simulink model "SimulacionControlador"  (R2023a)
settings: Solver=VariableStepAuto  StartTime=0.0  StopTime=5.0  RelTol=1e-3
settings Model: Creator=camil  LastModifiedBy=daniv

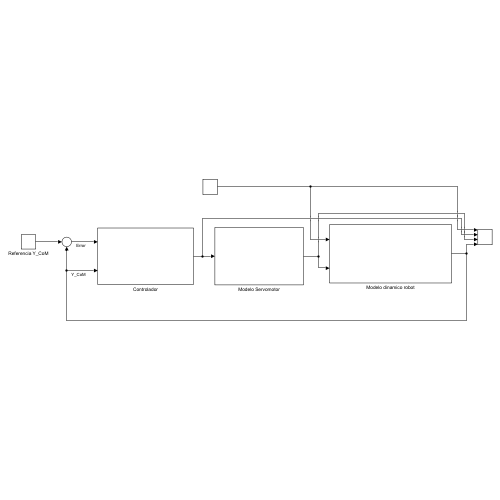
[thumbnail: Simulink's stored preview of the top-level diagram]
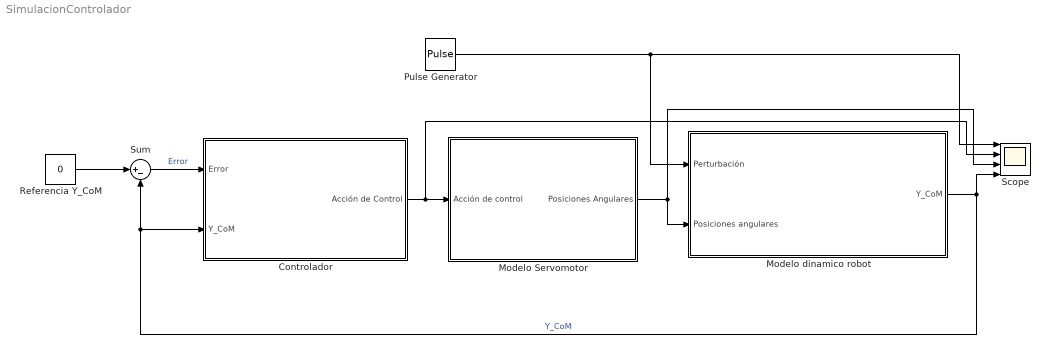
== system SimulacionControlador ==
  Controlador : Subsystem
  Modelo Servomotor : Subsystem
  Modelo dinamico robot : Subsystem
  Pulse Generator : DiscretePulseGenerator  PulseType=Time based  Amplitude=20  PulseWidth=50  PhaseDelay=1
  Referencia Y_CoM : Constant  Value=0
  Scope : Scope  NumInputPorts=4
  Sum : Sum  Inputs=|+-
  wires:
  Referencia Y_CoM/1 -> Sum/1
  Modelo Servomotor/1(Posiciones Angulares) -> Scope/3, Modelo dinamico robot/2(Posiciones angulares)
  Pulse Generator/1 -> Scope/1, Modelo dinamico robot/1(Perturbación)
  Controlador/1(Acción de Control) -> Scope/2, Modelo Servomotor/1(Acción de control)
  Sum/1 -> Controlador/1(Error)  "Error"
  Modelo dinamico robot/1(Y_CoM) -> Sum/2, Controlador/2(Y_CoM), Scope/4  "Y_CoM"

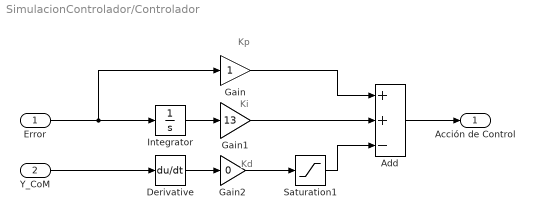
== system SimulacionControlador/Controlador ==
  note: Kd
  note: Ki
  note: Kp
  Error : Inport
  Y_CoM : Inport  Port=2
  Add : Sum  Inputs=++-
  Derivative : Derivative
  Gain : Gain
  Gain1 : Gain  Gain=13
  Gain2 : Gain  Gain=0
  Integrator : Integrator
  Saturation1 : Saturate  UpperLimit=10  LowerLimit=-10
  Acción de Control : Outport
  wires:
  Derivative/1 -> Gain2/1
  Add/1 -> Acción de Control/1
  Error/1 -> Integrator/1, Gain/1
  Saturation1/1 -> Add/3
  Gain/1 -> Add/1
  Gain1/1 -> Add/2
  Integrator/1 -> Gain1/1
  Y_CoM/1 -> Derivative/1
  Gain2/1 -> Saturation1/1

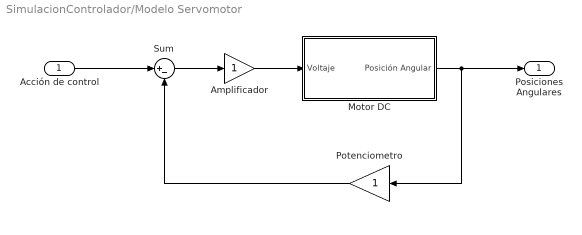
== system SimulacionControlador/Modelo Servomotor ==
  Acción de control : Inport
  Amplificador : Gain
  Motor DC : Subsystem
  Potenciometro : Gain
  Sum : Sum  Inputs=|+-
  Posiciones Angulares : Outport
  wires:
  Motor DC/1(Posición Angular) -> Posiciones Angulares/1, Potenciometro/1
  Acción de control/1 -> Sum/1
  Sum/1 -> Amplificador/1
  Potenciometro/1 -> Sum/2
  Amplificador/1 -> Motor DC/1(Voltaje)

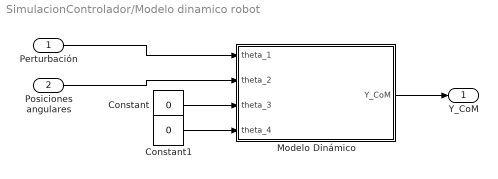
== system SimulacionControlador/Modelo dinamico robot ==
  Perturbación : Inport
  Posiciones angulares : Inport  Port=2
  Constant : Constant  Value=0
  Constant1 : Constant  Value=0
  Modelo Dinámico : MATLAB Function  TreatAsAtomicUnit=on
  Y_CoM : Outport
  wires:
  Perturbación/1 -> Modelo Dinámico/1(theta_1)
  Constant1/1 -> Modelo Dinámico/4(theta_4)
  Constant/1 -> Modelo Dinámico/3(theta_3)
  Modelo Dinámico/1(Y_CoM) -> Y_CoM/1
  Posiciones angulares/1 -> Modelo Dinámico/2(theta_2)

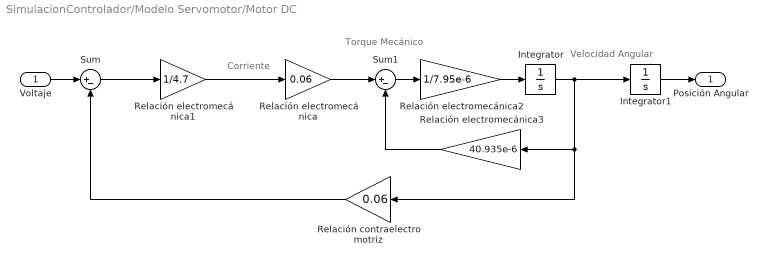
== system SimulacionControlador/Modelo Servomotor/Motor DC ==
  note: Torque
      | Mecánico
  note: Corriente
  note: Velocidad
      | Angular
  Voltaje : Inport
  Integrator : Integrator
  Integrator1 : Integrator
  Relación contraelectromotriz : Gain  Gain=0.06
  Relación electromecánica : Gain  Gain=0.06
  Relación electromecánica1 : Gain  Gain=1/4.7
  Relación electromecánica2 : Gain  Gain=1/7.95e-6
  Relación electromecánica3 : Gain  Gain=40.935e-6
  Sum : Sum  Inputs=|+-
  Sum1 : Sum  Inputs=|+-
  Posición Angular : Outport
  wires:
  Relación electromecánica3/1 -> Sum1/2
  Relación electromecánica2/1 -> Integrator/1
  Sum1/1 -> Relación electromecánica2/1
  Sum/1 -> Relación electromecánica1/1
  Relación electromecánica1/1 -> Relación electromecánica/1
  Relación contraelectromotriz/1 -> Sum/2
  Integrator/1 -> Integrator1/1, Relación electromecánica3/1, Relación contraelectromotriz/1
  Relación electromecánica/1 -> Sum1/1
  Voltaje/1 -> Sum/1
  Integrator1/1 -> Posición Angular/1

== matlab function SimulacionControlador/Modelo dinamico robot/Modelo Dinámico ==
  data: theta_1 input; Y_CoM output; theta_2 input; theta_3 input; theta_4 input
function Y_CoM = fcn(theta_1, theta_2, theta_3, theta_4)

% Vector de posiciones angulares
theta = [theta_1, theta_2, theta_3, theta_4];

% Vector de longitudes
L = [4, 24.5, 29, 11];

% Vector de posiciones de articulaciones
x = [0, 0, 0, 0];

% Calculo de posiciones de articulaciones
theta_sum = 0;
x_ant = 0;
for i = 1:length(theta)
        
    %Posicion x anterior
    if i == 1
        x_ant = 0;
    else 
        x_ant = x(i-1);
    end
    
    %Sumatoria de angulos
    for j = 1:i
        theta_sum = theta_sum + theta(i);
    end
    
    x(i) = x_ant + L(i)*sin((pi*theta_sum)/180);
end

% Vector de pesos
weight = [500, 334, 500, 330];

% Centro de masa
Y_CoM = 0;

% Calculo centro de masa

M_t = sum(weight);
for i = 1:length(x)
    Y_CoM = Y_CoM + x(i)*weight(i);
end

Y_CoM = Y_CoM/M_t;
